simulink model "signalsKF"  (R2021b)
settings: Solver=VariableStepAuto  StartTime=0.0  StopTime=10.0  RelTol=1e-3
undefined symbols (not defined in the file): sigbuilder_block
libraries: simulink x3
settings Model: Creator=riccardo  LastModifiedBy=buse

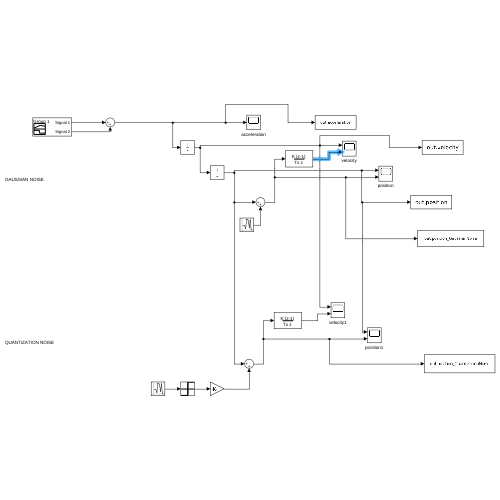
[thumbnail: Simulink's stored preview of the top-level diagram]
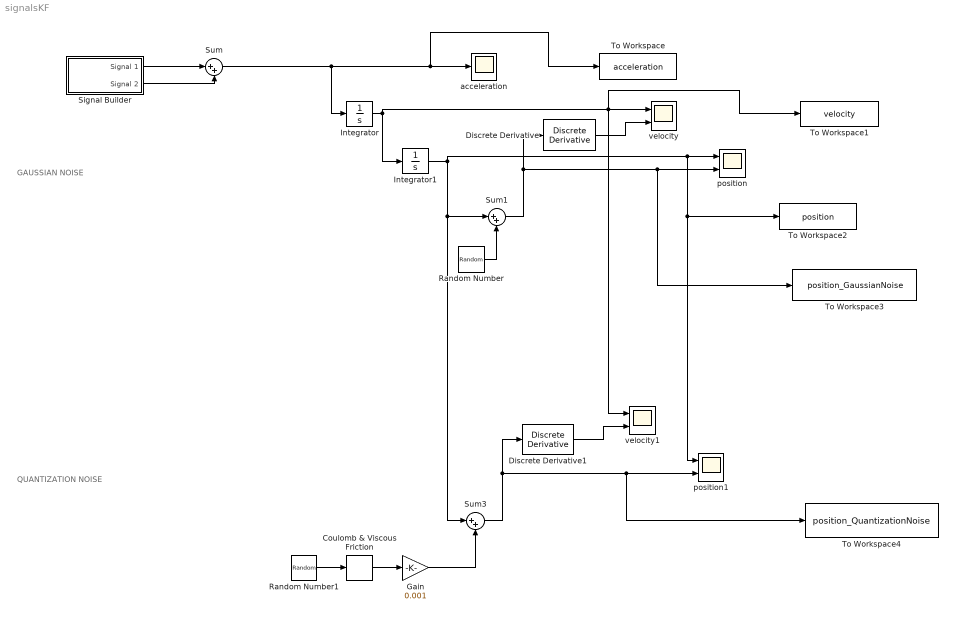
== system signalsKF ==
  note: GAUSSIAN NOISE
  note: QUANTIZATION NOISE
  Coulomb & Viscous Friction : simulink/Discontinuities/Coulomb & Viscous Friction  offset=[1]  gain=0
  Discrete Derivative : simulink/Discrete/Discrete Derivative  gainval=1  ICPrevScaledInput=0.0  OutMin=[]  OutMax=[]  OutDataType=fixdt(1, 16)  OutScaling=2^-10  DoSatur=off
  Discrete Derivative1 : simulink/Discrete/Discrete Derivative  gainval=1  ICPrevScaledInput=0.0  OutMin=[]  OutMax=[]  OutDataType=fixdt(1, 16)  OutScaling=2^-10  DoSatur=off
  Gain : Gain  Gain=0.001
  Integrator : Integrator
  Integrator1 : Integrator
  Random Number : RandomNumber  Variance=0.000001  SampleTime=0.001
  Random Number1 : RandomNumber  Variance=0.0001  SampleTime=0.001
  Signal Builder : Subsystem  Tag=STV Subsys  LoadFcn=sigbuilder_block('load');  StartFcn=sigbuilder_block('start');  StopFcn=sigbuilder_block('stop');  ClipboardFcn=sigbuilder_block('clipboard');  mask(Sigbuilder block){tuvar=[0:10]}
      mask help: Simulink:masks:SigbuilderBlock_MD
      mask init:
      | if ~strcmp(get_param(bdroot(gcbh),'SimulationStatus'),'stopped') tuvar = sigbuilder_block('maskInit'); end
      settings: CopyFcn=sigbuilder_block('copy');  DeleteFcn=sigbuilder_block('delete');  ModelCloseFcn=sigbuilder_block('modelClose');  PreSaveFcn=sigbuilder_block('preSave');  PauseFcn=sigbuilder_block('pause');  ContinueFcn=sigbuilder_block('continue');  NameChangeFcn=sigbuilder_block('namechange');  OpenFcn=sigbuilder_block('open',[437.6 194.25 542.65 404.95 ]);  CloseFcn=sigbuilder_block('close');
      mask Display: plot(0, 0, 100, 100,[2, 2, 32, 32, 2], [68, 8, 8, 68, 68],[32, 2], [38, 38], [32, 19, 2],[53, 60, 44], [32, 17, 17, 2],[16, 16, 31, 31]);txt = getActiveGroup(gcbh);text(2, 100, txt,'verticalAlignment', 'top');
  Sum : Sum  Inputs=|++
  Sum1 : Sum  Inputs=|++
  Sum3 : Sum  Inputs=|++
  To Workspace : ToWorkspace  VariableName=acceleration  SaveFormat=Structure With Time  SampleTime=0.001
  To Workspace1 : ToWorkspace  VariableName=velocity  SaveFormat=Structure With Time  SampleTime=0.001
  To Workspace2 : ToWorkspace  VariableName=position  SaveFormat=Structure With Time  SampleTime=0.001
  To Workspace3 : ToWorkspace  VariableName=position_GaussianNoise  SaveFormat=Structure With Time  SampleTime=0.001
  To Workspace4 : ToWorkspace  VariableName=position_QuantizationNoise  SaveFormat=Timeseries  SampleTime=0.001
  acceleration : Scope
  position : Scope  NumInputPorts=2
  position1 : Scope  NumInputPorts=2
  velocity : Scope  NumInputPorts=2
  velocity1 : Scope  NumInputPorts=2
  wires:
  Signal Builder/1(Signal 1) -> Sum/1
  Signal Builder/2(Signal 2) -> Sum/2
  Integrator/1 -> Integrator1/1, velocity1/1, To Workspace1/1, velocity/1
  Integrator1/1 -> Sum3/1, Sum1/1, position1/1, To Workspace2/1, position/1
  Random Number/1 -> Sum1/2
  Sum1/1 -> To Workspace3/1, position/2, Discrete Derivative/1
  Discrete Derivative/1 -> velocity/2
  Discrete Derivative1/1 -> velocity1/2
  Sum/1 -> Integrator/1, To Workspace/1, acceleration/1
  Random Number1/1 -> Coulomb & Viscous Friction/1
  Sum3/1 -> To Workspace4/1, position1/2, Discrete Derivative1/1
  Coulomb & Viscous Friction/1 -> Gain/1
  Gain/1 -> Sum3/2

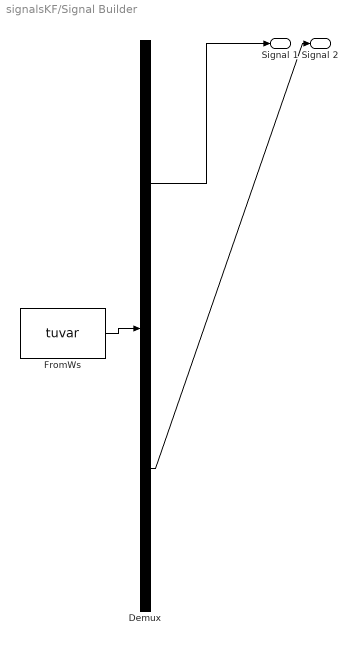
== system signalsKF/Signal Builder ==
  Demux : Demux  Tag=STV Demux  Outputs=2
      settings: DisplayOption=none
  FromWs : FromWorkspace  Tag=STV FromWs  VariableName=tuvar
      SigBuilderData=|
      | common.afterFinalStr = 'Extrapolate'
      | common.sampleTime = 0
      | dataSet.timeRange = [0 10]
      | dataSet.name = 'Group 1'
      | sbobj.Groups.Name = 'Group 1'
      | sbobj.Groups.Signals(1).Name = 'Signal 1'
      | sbobj.Groups.Signals(1).XData = [0 1 1 3 3 10]
      | sbobj.Groups.Signals(1).YData = [0 0 1 1 0 0]
      | sbobj.Groups.Signals(2).Name = 'Signal 2'
      | sbobj.Groups.Signals(2).XData = [0 7 7 9 9 10]
      | sbobj.Groups.Signals(2).YData = [0 0 -1 -1 0 0]
  Signal 1 : Outport  Tag=STV Outport
  Signal 2 : Outport  Tag=STV Outport  Port=2
  wires:
  Demux/1 -> Signal 1/1
  FromWs/1 -> Demux/1
  Demux/2 -> Signal 2/1
